simulink model "Projet_Final"  (R2024a)
settings: Solver=FixedStepAuto  StartTime=0.0  StopTime=6  FixedStep=Ts  RelTol=1e-3
values from neighbouring files (symbols this model uses):
  A1 = 0.548    [Parameters.m]
  A2 = 116    [Parameters.m]
  A3 = 0.4    [Parameters.m]
  A4 = 5    [Parameters.m]
  A5 = -21    [Parameters.m]
  A6 = 0.0068    [Parameters.m]
  C_Bat = 1e-3    (= 0.001)    [Parameters.m]    (also in Params_Battery_converter.m)
  C_dc = 4.5e-3    (= 0.0045)    [Parameters.m]
  f = 50    [Parameters.m]
  F = 0.0004924    [Parameters.m]
  G = 6.24    [Parameters.m]
  J = J_PMSG    (= 0.2227)    [Parameters.m]
  J_PMSG = 0.2227    [Parameters.m]
  ki_Ibat = 550    [Parameters.m]    (also in Params_Battery_converter.m)
  ki_id_grid = 225    [Parameters.m]
  ki_iq_grid = ki_id_grid    (= 225)    [Parameters.m]
  ki_isd = 13800    [Parameters.m]
  ki_omega = 0.6873    [Parameters.m]
  ki_PLL = 3200    [Parameters.m]
  ki_Q = 0.05    [Parameters.m]
  ki_vdc = C_dc * W_vdc^2    (= 28.8)    [Parameters.m]
  kp_Ibat = 6.28    [Parameters.m]    (also in Params_Battery_converter.m)
  kp_id_grid = 4.5    [Parameters.m]
  kp_iq_grid = kp_id_grid    (= 4.5)    [Parameters.m]
  kp_isd = 2.75    [Parameters.m]
  kp_omega = 3.108    [Parameters.m]
  kp_PLL = 180    [Parameters.m]
  kp_Q = 0.0005    [Parameters.m]
  kp_vdc = 2 * C_dc * W_vdc    (= 0.72)    [Parameters.m]
  Kt = 1.5 * p * Phi_r    (= 0.7164)    [Parameters.m]
  L_Bat = 2e-3    (= 0.002)    [Parameters.m]    (also in Params_Battery_converter.m)
  Lf = 8e-3    (= 0.008)    [Parameters.m]
  Ls = 0.000395    [Parameters.m]
  p = 4    [Parameters.m]
  Phi_r = 0.1194    [Parameters.m]
  R = 3.96    [Parameters.m]
  Rf = 0.01    [Parameters.m]
  rho = 1.225    [Parameters.m]
  Rs = 0.0485    [Parameters.m]
  S = pi*R^2    (= 49.2651993565)    [Parameters.m]
  Ts = 1e-6    (= 1e-06)    [Parameters.m]
  Vdc_ref = 700    [Parameters.m]    (also in Params_Battery_converter.m)
undefined symbols (not defined in the file or in its folder): Ion, Lithium
libraries: spsSeriesRLCBranchLib x19, slpidlib x11, spsMeanLib x6, spsThreePhaseVIMeasurementLib x6, spsThreePhaseBreakerLib x6, spsIdealSwitchLib x4, spsThreePhaseParallelRLCLoadLib x4, spsCurrentMeasurementLib x3, eeTransforms x3, spsPWMGenerator2LevelLib x3, spsVoltageMeasurementLib x3, spsUniversalBridgeLib x2
(part 2 of 3)

== system Projet_Final/Bidirectional DC–DC Converter/Battery Controller ==
  V_bat : Inport
  I_bat : Inport  Port=2
  P1 : Inport  Port=3
  P2 : Inport  Port=4
  Add2 : Sum  Inputs=+-
  Boucle I_bat : Scope  NumInputPorts=2
  Divide : Product  Inputs=*/
  PID Controller3 : slpidlib/PID Controller  Controller=PID  Form=Parallel  TimeDomain=Continuous-time  UseExternalTs=off  SampleTime=-1  IntegratorMethod=Forward Euler  FilterMethod=Forward Euler  ControllerParametersSource=internal  P=kp_Ibat  I=ki_Ibat  UseKiTs=off  D=0  UseExternalDerivativeSource=off  N=100  UseFilter=on  TunerSelectOption=Transfer Function Based (PID Tuner App)  InitialConditionSource=internal  InitialConditionForIntegrator=0  InitialConditionForFilter=0  DifferentiatorICPrevScaledInput=0  ExternalReset=none  TrackingMode=off  Kt=1  LimitOutput=off  SatLimitsSource=internal  UpperSaturationLimit=inf  LowerSaturationLimit=-inf  LinearizeAsGain=off  AntiWindupMode=none  Kb=1  LimitIntegrator=off  UpperIntegratorSaturationLimit=inf  LowerIntegratorSaturationLimit=-inf  POutMin=[]  POutMax=[]  IOutMin=[]  IOutMax=[]  DOutMin=[]  DOutMax=[]  NOutMin=[]  NOutMax=[]  SumOutMin=[]  SumOutMax=[]  SaturationOutMin=[]  SaturationOutMax=[]  PParamMin=[]  PParamMax=[]  IParamMin=[]  IParamMax=[]  DParamMin=[]  DParamMax=[]  NParamMin=[]  NParamMax=[]  KbParamMin=[]  KbParamMax=[]  KtParamMin=[]  KtParamMax=[]  KbOutMin=[]  KbOutMax=[]  KtOutMin=[]  KtOutMax=[]  IntegratorOutMin=[]  IntegratorOutMax=[]  FilterOutMin=[]  FilterOutMax=[]  SumI1OutMin=[]  SumI1OutMax=[]  SumI2OutMin=[]  SumI2OutMax=[]  SumI3OutMin=[]  SumI3OutMax=[]  SumI4OutMin=[]  SumI4OutMax=[]  SumDOutMin=[]  SumDOutMax=[]  DifferentiatorOutMin=[]  DifferentiatorOutMax=[]  FilterDiffOutCoefMin=[]  FilterDiffOutCoefMax=[]  ReciprocalOutMin=[]  ReciprocalOutMax=[]  SumDenOutMin=[]  SumDenOutMax=[]  SumNumOutMin=[]  SumNumOutMax=[]  DivideOutMin=[]  DivideOutMax=[]  UdiffTsProdOutMin=[]  UdiffTsProdOutMax=[]  NTsProdOutMin=[]  NTsProdOutMax=[]  UintegralTsProdOutMin=[]  UintegralTsProdOutMax=[]  UngainTsProdOutMin=[]  UngainTsProdOutMax=[]  ClampingZeroOutDataTypeStr=Inherit: Inherit via back propagation  ClampingZeroOutMin=[]  ClampingZeroOutMax=[]  FilterDenConstantOutDataTypeStr=Inherit: Inherit via back propagation  FilterDenConstantOutMin=[]  FilterDenConstantOutMax=[]  PCopyOutDataTypeStr=Inherit: Inherit via back propagation  PCopyOutMin=[]  PCopyOutMax=[]  NCopyOutDataTypeStr=Inherit: Inherit via back propagation  NCopyOutMin=[]  NCopyOutMax=[]  IntegratorContinuousStateAttributes=''  IntegratorStateMustResolveToSignalObject=off  IntegratorRTWStateStorageClass=Auto  FilterContinuousStateAttributes=''  FilterStateMustResolveToSignalObject=off  FilterRTWStateStorageClass=Auto  ParallelPVariant=InternalParameters  IdealPVariant=Disabled  IVariant=InternalParameters  DVariant=InternalParameters  IntegratorVariant=Continuous  SatVariant=Disabled  AWVariant=Passthrough  PCopyVariant=Disabled  TRVariant=Disabled  FdbkBlocksVariant=Forward  IdealPFdbkVariant=Disabled  SatFdbkVariant=Disabled  DerivativeFilterVariant=ContFilter  NVariant=InternalParameters  NCopyVariant=Disabled  FilterICVariant=InternalICsFilter  IntegratorICVariant=InternalICs  ExternalResetVariant=Disabled  TRSumVariant=Passthrough  SumFdbkVariant=Disabled  SumVariant=Sum_PID  TsampFilterVariant=InternalTs  TsampNgainVariant=Passthrough  TsampIntegralVariant=Disabled_SignalSpec  ExternalSaturationOutDataTypeStr=Inherit: Same as second input  DerivativeSourceVariant=ErrorSignal
  PWM Generator_ Single phase Half Bridge : Subsystem
  Saturation1 : Saturate  UpperLimit=700  LowerLimit=0.001
  Sum : Sum  Inputs=-+|
  Transfer Fcn3 : TransferFcn  Denominator=[1e-6 1]
  Transfer Fcn4 : TransferFcn  Denominator=[1e-6 1]
  PWM_1 : Outport  OutputWhenDisabled=reset  InitialOutput=0  VectorParamsAs1DForOutWhenUnconnected=off
  PWM_2 : Outport  Port=2  OutputWhenDisabled=reset  InitialOutput=0  VectorParamsAs1DForOutWhenUnconnected=off
  wires:
  I_bat/1 -> Transfer Fcn4/1
  PWM Generator_ Single phase Half Bridge/1(Buck) -> PWM_1/1
  PWM Generator_ Single phase Half Bridge/2(Boost) -> PWM_2/1
  PID Controller3/1 -> PWM Generator_ Single phase Half Bridge/1(err_filter)
  Sum/1 -> Transfer Fcn3/1
  Divide/1 -> Sum/2, Boucle I_bat/1
  Transfer Fcn3/1 -> PID Controller3/1
  Transfer Fcn4/1 -> Sum/1, Boucle I_bat/2
  Saturation1/1 -> Divide/2
  Add2/1 -> Divide/1
  V_bat/1 -> Saturation1/1
  P1/1 -> Add2/1
  P2/1 -> Add2/2

== system Projet_Final/Residential Load/Subsystem ==
  Constant2 : Constant
  Step : Step  Time=2  SampleTime=0
  Step1 : Step  Time=4  SampleTime=0
  tag scope: Charge1_ON=global, Charge2_ON=global, Charge3_ON=global
  wires:
  Constant2/1 -> [Charge1_ON]
  Step/1 -> [Charge2_ON]
  Step1/1 -> [Charge3_ON]

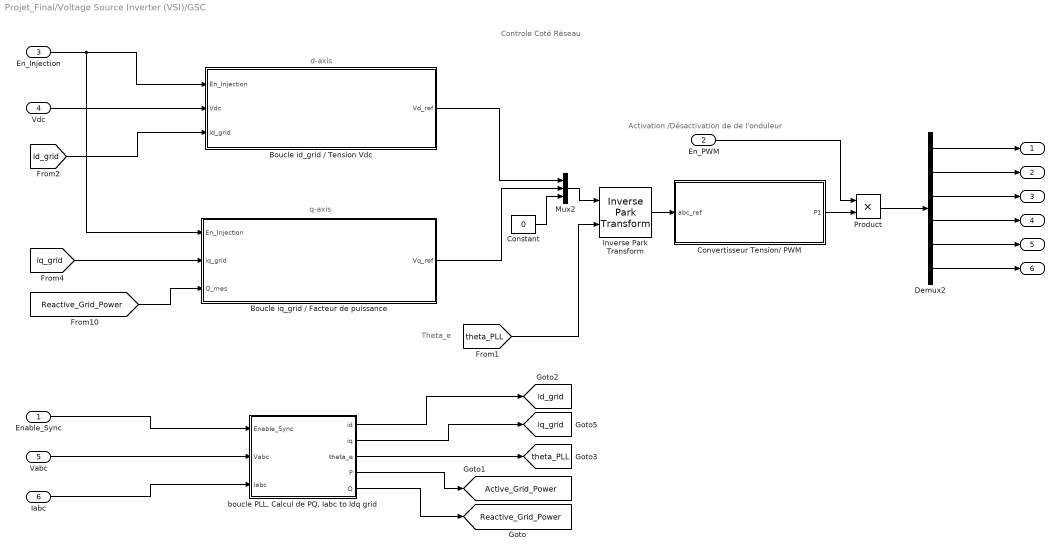
== system Projet_Final/Voltage Source Inverter (VSI)/GSC ==
  note: Controle Coté Réseau
  note: Activation /Désactivation de de l'onduleur
  note: d-axis
  note: Theta_e
  note: q-axis
  Enable_Sync : Inport
  En_PWM : Inport  Port=2
  En_Injection : Inport  Port=3
  Vdc : Inport  Port=4
  Vabc : Inport  Port=5
  Iabc : Inport  Port=6
  Boucle id_grid / Tension Vdc : Subsystem
  Boucle iq_grid / Facteur de puissance : Subsystem
  Constant : Constant  Value=0
  "Convertisseur Tension/ PWM " : Subsystem
  Demux2 : Demux  Outputs=6
  Inverse Park Transform : eeTransforms/Inverse Park Transform  AxisAlignment=Q-axis  PowerInvariant=off
      settings: LibrarySourceBlock=|
      | ee_sl_lib/Mathematical
      | Transforms/Inverse
      | Park Transform
  Mux2 : Mux  Inputs=3
  Product : Product
  "boucle PLL, Calcul de PQ, Iabc to Idq grid" : Subsystem
  " " : Outport
  "  " : Outport  Port=2
  "   " : Outport  Port=3
  "    " : Outport  Port=4
  "     " : Outport  Port=5
  "      " : Outport  Port=6
  tag scope: Active_Grid_Power=global, Reactive_Grid_Power=global, id_grid=global, iq_grid=global, theta_PLL=global
  wires:
  Mux2/1 -> Inverse Park Transform/1
  Constant/1 -> Mux2/3
  Inverse Park Transform/1 -> "Convertisseur Tension/ PWM "/1(abc_ref)
  Boucle iq_grid / Facteur de puissance/1(Vq_ref) -> Mux2/2
  Boucle id_grid / Tension Vdc/1(Vd_ref) -> Mux2/1
  Demux2/6 -> "      "/1
  Product/1 -> Demux2/1
  Demux2/3 -> "   "/1
  Demux2/5 -> "     "/1
  Demux2/1 -> " "/1
  Demux2/4 -> "    "/1
  Demux2/2 -> "  "/1
  "Convertisseur Tension/ PWM "/1(P1) -> Product/2
  Vdc/1 -> Boucle id_grid / Tension Vdc/2(Vdc)
  [id_grid] -> Boucle id_grid / Tension Vdc/3(id_grid)
  [Reactive_Grid_Power] -> Boucle iq_grid / Facteur de puissance/3(Q_mes)
  [iq_grid] -> Boucle iq_grid / Facteur de puissance/2(iq_grid)
  [theta_PLL] -> Inverse Park Transform/2
  Vabc/1 -> "boucle PLL, Calcul de PQ, Iabc to Idq grid"/2(Vabc)
  Iabc/1 -> "boucle PLL, Calcul de PQ, Iabc to Idq grid"/3(Iabc)
  "boucle PLL, Calcul de PQ, Iabc to Idq grid"/5(Q) -> [Reactive_Grid_Power]
  "boucle PLL, Calcul de PQ, Iabc to Idq grid"/4(P) -> [Active_Grid_Power]
  "boucle PLL, Calcul de PQ, Iabc to Idq grid"/1(id) -> [id_grid]
  "boucle PLL, Calcul de PQ, Iabc to Idq grid"/2(iq) -> [iq_grid]
  "boucle PLL, Calcul de PQ, Iabc to Idq grid"/3(theta_e) -> [theta_PLL]
  En_PWM/1 -> Product/1
  En_Injection/1 -> Boucle iq_grid / Facteur de puissance/1(En_Injection), Boucle id_grid / Tension Vdc/1(En_Injection)
  Enable_Sync/1 -> "boucle PLL, Calcul de PQ, Iabc to Idq grid"/1(Enable_Sync)

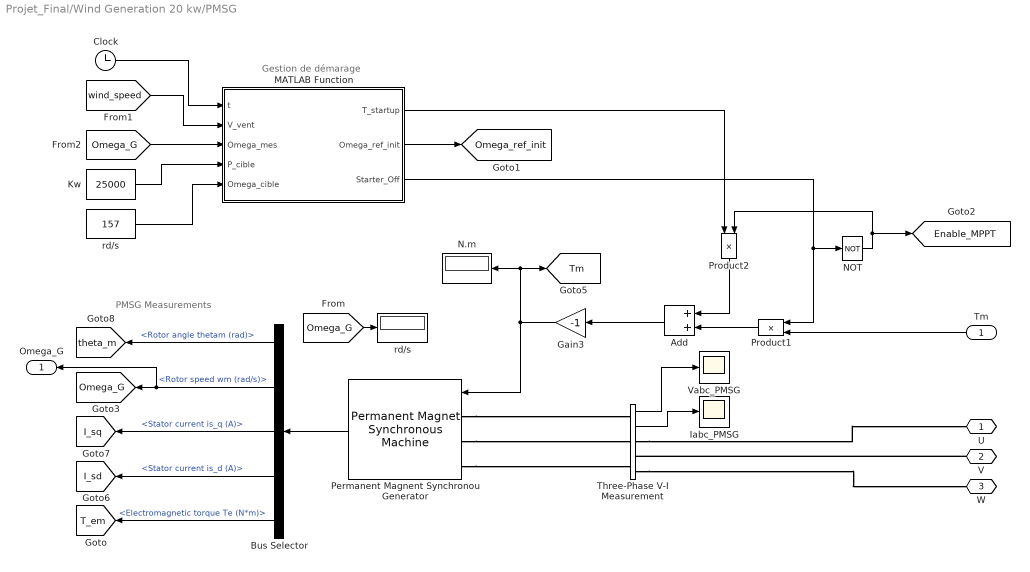
== system Projet_Final/Wind Generation 20 kw/PMSG ==
  note: Gestion de démarage
  note: PMSG Measurements
  Tm : Inport
  Add : Sum
  Bus Selector : BusSelector  OutputSignals=Rotor angle thetam (rad),Rotor speed wm (rad/s),Stator current is_q (A),Stator current is_d (A),Electromagnetic torque Te (N*m)
  Clock : Clock
  Gain3 : Gain  Gain=-1
  Iabc_PMSG : Scope
  Kw : Constant  Value=25000
  MATLAB Function : MATLAB Function  TreatAsAtomicUnit=on  SystemSampleTime=Ts
  N.m : Display
      settings: Format=bank
  NOT : Logic  Operator=NOT  IconShape=distinctive  AllPortsSameDT=off  OutDataTypeStr=boolean
  Permanent Magnent Synchronou Generator : spsPermanentMagnetSynchronousMachineLib/Permanent Magnet Synchronous Machine  NbPhases=3  FluxDistribution=Sinusoidal  RotorType=Round  MechanicalLoad=Torque Tm  PresetModel=No  ShowDetailedParameters=on  MeasurementBus=off  Resistance=Rs  Inductance=8.5e-3  dqInductances=[8.5e-3,8.5e-3]  La=Ls  MachineConstant=Flux linkage established by magnets (V.s)  Flux=Phi_r  VoltageCst=86.6271  TorqueCst=0.7164  Flat=120  Mechanical=[J F p 0]  PolePairs=4  InitialConditions=[0.01 ,0, 0,0]  InitialConditions5ph=[0 0 0 0 0 0]  RefAngle=90 degrees behind phase A axis (modified Park)  IterativeDiscreteModel=Trapezoidal non iterative  TsBlock=-1  TsPowergui=0
  Product1 : Product
  Product2 : Product
  Three-Phase V-I Measurement : spsThreePhaseVIMeasurementLib/Three-Phase V-I Measurement  VoltageMeasurement=phase-to-ground  SetLabelV=off  LabelV=Vabc  Vpu=off  VpuLL=off  CurrentMeasurement=yes  SetLabelI=off  LabelI=Iabc  Ipu=off  Pbase=100e6  Vbase=500e3  OutputType=Complex  PhasorSimulation=off  PSBequivalent=0
  Vabc_PMSG : Scope
  rd/s : Display
      settings: Format=bank
  "rd/s " : Constant  Value=157
  U : PMIOPort  Side=Right
  V : PMIOPort  Port=2  Side=Right
  W : PMIOPort  Port=3  Side=Right
  Omega_G : Outport
  tag scope: Enable_MPPT=global, I_sd=global, I_sq=global, Omega_G=global, Omega_ref_init=global, T_em=global, Tm=global, theta_m=global
  wires:
  Bus Selector/1 -> [theta_m]  "<Rotor angle thetam (rad)>"
  Bus Selector/2 -> Omega_G/1, [Omega_G]  "<Rotor speed wm (rad/s)>"
  Permanent Magnent Synchronou Generator/1 -> Bus Selector/1
  Bus Selector/4 -> [I_sd]  "<Stator current is_d (A)>"
  Bus Selector/5 -> [T_em]  "<Electromagnetic torque Te (N*m)>"
  Bus Selector/3 -> [I_sq]  "<Stator current is_q (A)>"
  Three-Phase V-I Measurement/1 -> Vabc_PMSG/1
  Three-Phase V-I Measurement/2 -> Iabc_PMSG/1
  Product1/1 -> Add/2
  MATLAB Function/3(Starter_Off) -> Product1/1, NOT/1
  MATLAB Function/2(Omega_ref_init) -> [Omega_ref_init]
  MATLAB Function/1(T_startup) -> Product2/1
  [Omega_G] -> MATLAB Function/3(Omega_mes)
  NOT/1 -> [Enable_MPPT], Product2/2
  [wind_speed] -> MATLAB Function/2(V_vent)
  Product2/1 -> Add/1
  Kw/1 -> MATLAB Function/4(P_cible)
  "rd/s "/1 -> MATLAB Function/5(Omega_cible)
  Clock/1 -> MATLAB Function/1(t)
  Add/1 -> Gain3/1
  Tm/1 -> Product1/2
  [Omega_G] -> rd/s/1
  Gain3/1 -> Permanent Magnent Synchronou Generator/1, [Tm], N.m/1
  connections:
  Permanent Magnent Synchronou Generator/LConn1 -- Three-Phase V-I Measurement/LConn1
  Permanent Magnent Synchronou Generator/LConn2 -- Three-Phase V-I Measurement/LConn2
  Permanent Magnent Synchronou Generator/LConn3 -- Three-Phase V-I Measurement/LConn3
  Three-Phase V-I Measurement/RConn1 -- U/RConn1
  V/RConn1 -- Three-Phase V-I Measurement/RConn2
  Three-Phase V-I Measurement/RConn3 -- W/RConn1

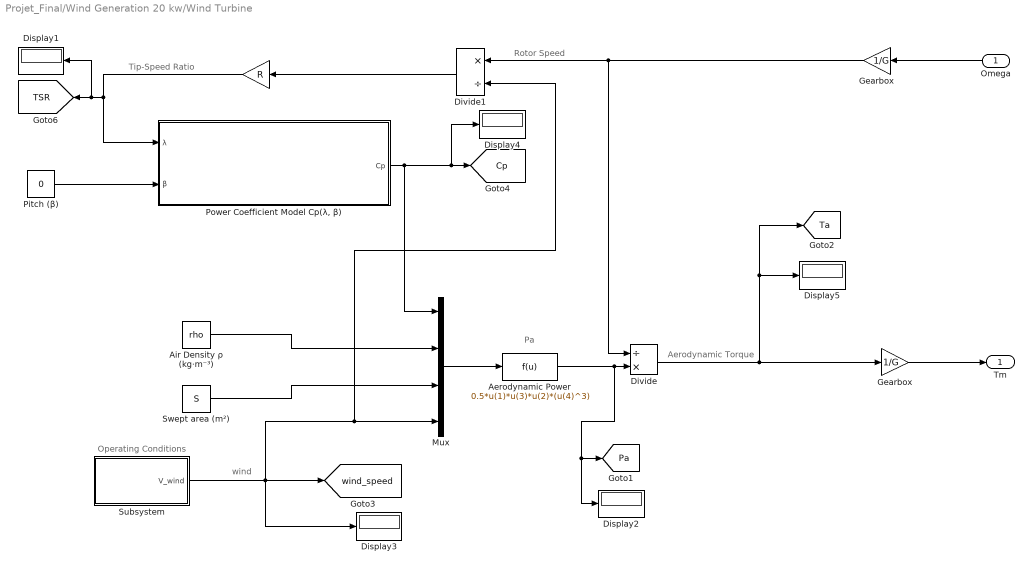
== system Projet_Final/Wind Generation 20 kw/Wind Turbine ==
  note: wind
  note: Rotor Speed
  note: Aerodynamic Torque
  note: Pa
  note: Operating Conditions
  note: Tip-Speed Ratio
  Omega : Inport
  "   " : Gain  Gain=R
  "Aerodynamic Power " : Fcn  Expr=0.5*u(1)*u(3)*u(2)*(u(4)^3)
  Air Density ρ (kg·m⁻³) : Constant  Value=rho
  Display{1..5} (5 alike) : Display
      settings: Format=bank
  Divide : Product  Inputs=/*
  Divide1 : Product  Inputs=*/
  Gearbox : Gain  Gain=1/G
  "Gearbox   " : Gain  Gain=1/G
  Mux : Mux
  "Pitch (β) " : Constant  Value=0
  "Power Coefficient Model Cp(λ, β)" : Subsystem
  Subsystem : Subsystem
  Swept area (m²) : Constant  Value=S
  Tm : Outport
  tag scope: Cp=global, Pa=global, TSR=global, Ta=global, wind_speed=global
  wires:
  Swept area (m²)/1 -> Mux/3
  "Power Coefficient Model Cp(λ, β)"/1(Cp) -> Display4/1, [Cp], Mux/1
  Subsystem/1(V_wind) -> Divide1/2, Mux/4, [wind_speed], Display3/1
  "Pitch (β) "/1 -> "Power Coefficient Model Cp(λ, β)"/2(β)
  Gearbox/1 -> Divide1/1, Divide/1
  Air Density ρ (kg·m⁻³)/1 -> Mux/2
  "   "/1 -> "Power Coefficient Model Cp(λ, β)"/1(λ), Display1/1, [TSR]
  Divide1/1 -> "   "/1
  Mux/1 -> "Aerodynamic Power "/1
  "Aerodynamic Power "/1 -> Display2/1, [Pa], Divide/2
  Divide/1 -> [Ta], Display5/1, "Gearbox   "/1
  "Gearbox   "/1 -> Tm/1
  Omega/1 -> Gearbox/1

== system Projet_Final/Active Rectifier/MSC/PWM Generation ==
  abc_ref : Inport
  Divide3 : Product  Inputs=*/
  PWM Generator (2-Level) : spsPWMGenerator2LevelLib/PWM Generator (2-Level)  ModulatorType=Three-phase bridge (6 pulses)  ModulatorMode=Unsynchronized  Fc=Fc  Pc=90  nF=27  MinMax="[ -1  1 ]"  SamplingTechnique=Natural  ModulatingSignals=off  m=0.8  Freq=60  Phase=0  Ts=Ts  ShowCarrierOutport=off
  Scope : Scope
  Unit Delay1 : UnitDelay  SampleTime=Ts  HasFrameUpgradeWarning=on
  indiceM=33_(1/(fr*33)3 : Constant  Value=Vdc_ref/2
  Commandes de Redresseur : Outport
  wires:
  indiceM=33_(1/(fr*33)3/1 -> Divide3/2
  abc_ref/1 -> Divide3/1
  PWM Generator (2-Level)/1 -> Commandes de Redresseur/1
  Unit Delay1/1 -> PWM Generator (2-Level)/1, Scope/1
  Divide3/1 -> Unit Delay1/1

== system Projet_Final/Active Rectifier/MSC/d-axis current controller with cross-coupling compensation ==
  note: isd_ref
  I_sd : Inport
  " Vd/Vdref" : Scope
  Constant : Constant  Value=0
  Decoupling Feedforward Terms : Subsystem
      settings: PortSchema="{\"entries\":[{\"content\":{\"sides\":[{\"content\":{\"connectorIds\":[\"In1\"]},\"type\":\"ConnectorPlacement.EquallySpacedRectSide\",\"uuid\":\"a35b541f-6c91-4579-89f1-6689e9beed7f\"},{\"content\":{\"connectorIds\":[\"Out1\"],\"side\":\"RIGHT\"},\"type\":\"ConnectorPlacement.EquallySpacedRectSide\",\"uuid\":\"c874527c-990c-4788-aa16-7f8a0c94d194\"},{\"content\":{\"side\":\"TOP\"},\"type\":\"ConnectorPlacement.EquallySpacedRectSide\",\"uuid\":\"b0161d26-106e-466a-8756-17981005591c\"},{\"content\":{\"connectorIds\":[\"In2\",\"In3\"],\"side\":\"BOTTOM\"},\"type\":\"ConnectorPlacement.EquallySpacedRectSide\",\"uuid\":\"87eba4bb-8cc6-4d91-843e-d033b71d377b\"}]},\"type\":\"ConnectorPlacement.EquallySpacedConnector\",\"uuid\":\"031ea5bd-d22b-4033-942a-a77822380b2b\"}],\"packageUris\":[\"http://schema.mathworks.com/mf0/Connector/R2020b\"],\"version\":\"1.0\"}"
  Mux1 : Mux  Inputs=2
  Mux2 : Mux  Inputs=2
  Sum : Sum  Inputs=+-
  Transfer Fcn{1..4} (4 alike) : TransferFcn  Denominator=[0.00004 1]
  d-axis Current Control Loop : Scope
  d-axis Current PI Controller : slpidlib/PID Controller  Controller=PI  Form=Parallel  TimeDomain=Continuous-time  UseExternalTs=off  SampleTime=Ts  IntegratorMethod=Forward Euler  FilterMethod=Forward Euler  ControllerParametersSource=internal  P=kp_isd  I=ki_isd  UseKiTs=off  D=0  UseExternalDerivativeSource=off  N=100  UseFilter=on  TunerSelectOption=Transfer Function Based (PID Tuner App)  InitialConditionSource=internal  InitialConditionForIntegrator=0  InitialConditionForFilter=0  DifferentiatorICPrevScaledInput=0  ExternalReset=none  TrackingMode=off  Kt=1  LimitOutput=off  SatLimitsSource=internal  UpperSaturationLimit=inf  LowerSaturationLimit=-inf  LinearizeAsGain=on  AntiWindupMode=none  Kb=1  LimitIntegrator=off  UpperIntegratorSaturationLimit=inf  LowerIntegratorSaturationLimit=-inf  POutMin=[]  POutMax=[]  IOutMin=[]  IOutMax=[]  DOutMin=[]  DOutMax=[]  NOutMin=[]  NOutMax=[]  SumOutMin=[]  SumOutMax=[]  SaturationOutMin=[]  SaturationOutMax=[]  PParamMin=[]  PParamMax=[]  IParamMin=[]  IParamMax=[]  DParamMin=[]  DParamMax=[]  NParamMin=[]  NParamMax=[]  KbParamMin=[]  KbParamMax=[]  KtParamMin=[]  KtParamMax=[]  KbOutMin=[]  KbOutMax=[]  KtOutMin=[]  KtOutMax=[]  IntegratorOutMin=[]  IntegratorOutMax=[]  FilterOutMin=[]  FilterOutMax=[]  SumI1OutMin=[]  SumI1OutMax=[]  SumI2OutMin=[]  SumI2OutMax=[]  SumI3OutMin=[]  SumI3OutMax=[]  SumI4OutMin=[]  SumI4OutMax=[]  SumDOutMin=[]  SumDOutMax=[]  DifferentiatorOutMin=[]  DifferentiatorOutMax=[]  FilterDiffOutCoefMin=[]  FilterDiffOutCoefMax=[]  ReciprocalOutMin=[]  ReciprocalOutMax=[]  SumDenOutMin=[]  SumDenOutMax=[]  SumNumOutMin=[]  SumNumOutMax=[]  DivideOutMin=[]  DivideOutMax=[]  UdiffTsProdOutMin=[]  UdiffTsProdOutMax=[]  NTsProdOutMin=[]  NTsProdOutMax=[]  UintegralTsProdOutMin=[]  UintegralTsProdOutMax=[]  UngainTsProdOutMin=[]  UngainTsProdOutMax=[]  ClampingZeroOutDataTypeStr=Inherit: Inherit via back propagation  ClampingZeroOutMin=[]  ClampingZeroOutMax=[]  FilterDenConstantOutDataTypeStr=Inherit: Inherit via back propagation  FilterDenConstantOutMin=[]  FilterDenConstantOutMax=[]  PCopyOutDataTypeStr=Inherit: Inherit via back propagation  PCopyOutMin=[]  PCopyOutMax=[]  NCopyOutDataTypeStr=Inherit: Inherit via back propagation  NCopyOutMin=[]  NCopyOutMax=[]  IntegratorContinuousStateAttributes=''  IntegratorStateMustResolveToSignalObject=off  IntegratorRTWStateStorageClass=Auto  FilterContinuousStateAttributes=''  FilterStateMustResolveToSignalObject=off  FilterRTWStateStorageClass=Auto  ParallelPVariant=InternalParameters  IdealPVariant=Disabled  IVariant=InternalParameters  DVariant=Disabled  IntegratorVariant=Continuous  SatVariant=Disabled  AWVariant=Passthrough  PCopyVariant=Disabled  TRVariant=Disabled  FdbkBlocksVariant=Forward  IdealPFdbkVariant=Disabled  SatFdbkVariant=Disabled  DerivativeFilterVariant=Disabled  NVariant=Disabled  NCopyVariant=Disabled_SignalSpec  FilterICVariant=Disabled  IntegratorICVariant=InternalICs  ExternalResetVariant=Disabled  TRSumVariant=Passthrough  SumFdbkVariant=Disabled  SumVariant=Sum_PI  TsampFilterVariant=InternalTs  TsampNgainVariant=Passthrough  TsampIntegralVariant=Disabled_SignalSpec  ExternalSaturationOutDataTypeStr=Inherit: Same as second input  DerivativeSourceVariant=Disabled
  Vd_ref : Outport
  wires:
  I_sd/1 -> Transfer Fcn4/1
  [I_sq] -> Transfer Fcn2/1
  [Omega_G] -> Decoupling Feedforward Terms/3(Wm)
  Mux1/1 -> d-axis Current Control Loop/1
  Constant/1 -> Sum/1, Mux1/2
  Sum/1 -> Transfer Fcn3/1
  Decoupling Feedforward Terms/1(Vdref) -> Mux2/2, Vd_ref/1
  d-axis Current PI Controller/1 -> Transfer Fcn1/1, Mux2/1
  Transfer Fcn2/1 -> Decoupling Feedforward Terms/2(Iq)
  Mux2/1 -> " Vd/Vdref"/1
  Transfer Fcn3/1 -> d-axis Current PI Controller/1
  Transfer Fcn1/1 -> Decoupling Feedforward Terms/1(vd)
  Transfer Fcn4/1 -> Sum/2, Mux1/1

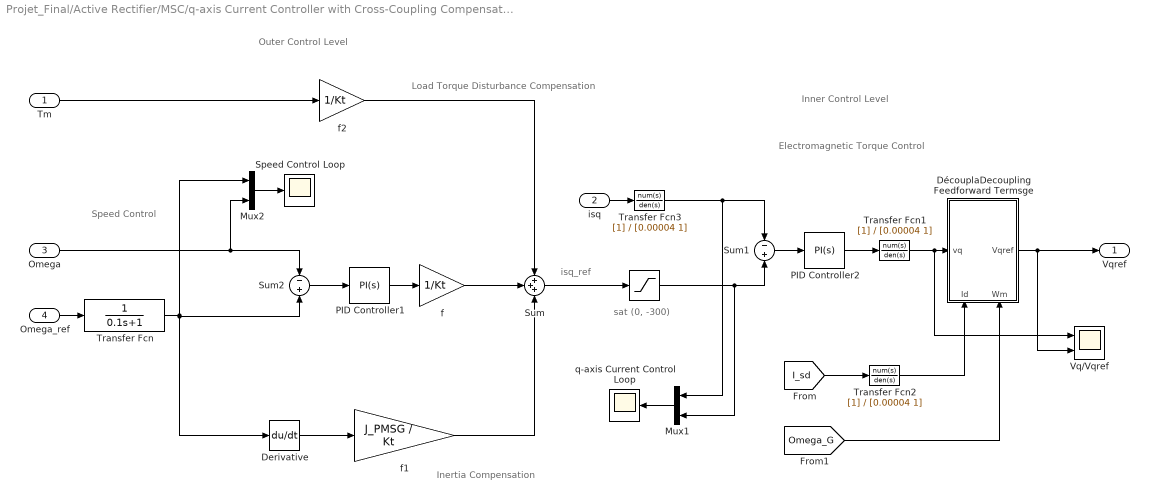
== system Projet_Final/Active Rectifier/MSC/q-axis Current Controller with Cross-Coupling Compensation  ==
  note: Speed Control
  note: sat (0, -300)
  note: Load Torque Disturbance Compensation
  note: isq_ref
  note: Inertia Compensation
  note: Electromagnetic Torque Control
  note: Inner Control Level
  note: Outer Control Level
  Tm : Inport
  isq : Inport  Port=2
  Omega : Inport  Port=3
  Omega_ref : Inport  Port=4
  "  " : Saturate  UpperLimit=0  LowerLimit=-300
  Derivative : Derivative
  DécouplaDecoupling Feedforward Termsge : Subsystem
      settings: PortSchema="{\"entries\":[{\"content\":{\"sides\":[{\"content\":{\"connectorIds\":[\"In1\"]},\"type\":\"ConnectorPlacement.EquallySpacedRectSide\",\"uuid\":\"a35b541f-6c91-4579-89f1-6689e9beed7f\"},{\"content\":{\"connectorIds\":[\"Out1\"],\"side\":\"RIGHT\"},\"type\":\"ConnectorPlacement.EquallySpacedRectSide\",\"uuid\":\"c874527c-990c-4788-aa16-7f8a0c94d194\"},{\"content\":{\"side\":\"TOP\"},\"type\":\"ConnectorPlacement.EquallySpacedRectSide\",\"uuid\":\"b0161d26-106e-466a-8756-17981005591c\"},{\"content\":{\"connectorIds\":[\"In2\",\"In3\"],\"side\":\"BOTTOM\"},\"type\":\"ConnectorPlacement.EquallySpacedRectSide\",\"uuid\":\"6bea0741-ba37-48dd-9c1f-2166530afd2a\"}]},\"type\":\"ConnectorPlacement.EquallySpacedConnector\",\"uuid\":\"031ea5bd-d22b-4033-942a-a77822380b2b\"}],\"packageUris\":[\"http://schema.mathworks.com/mf0/Connector/R2020b\"],\"version\":\"1.0\"}"
  Mux1 : Mux  Inputs=2
  Mux2 : Mux  Inputs=2
  PID Controller1 : slpidlib/PID Controller  Controller=PI  Form=Parallel  TimeDomain=Continuous-time  UseExternalTs=off  SampleTime=Ts  IntegratorMethod=Forward Euler  FilterMethod=Forward Euler  ControllerParametersSource=internal  P=kp_omega  I=ki_omega  UseKiTs=off  D=0  UseExternalDerivativeSource=off  N=100  UseFilter=on  TunerSelectOption=Transfer Function Based (PID Tuner App)  InitialConditionSource=internal  InitialConditionForIntegrator=0  InitialConditionForFilter=0  DifferentiatorICPrevScaledInput=0  ExternalReset=none  TrackingMode=off  Kt=1  LimitOutput=off  SatLimitsSource=internal  UpperSaturationLimit=222.3  LowerSaturationLimit=0  LinearizeAsGain=on  AntiWindupMode=back-calculation  Kb=1  LimitIntegrator=off  UpperIntegratorSaturationLimit=inf  LowerIntegratorSaturationLimit=-inf  POutMin=[]  POutMax=[]  IOutMin=[]  IOutMax=[]  DOutMin=[]  DOutMax=[]  NOutMin=[]  NOutMax=[]  SumOutMin=[]  SumOutMax=[]  SaturationOutMin=[]  SaturationOutMax=[]  PParamMin=[]  PParamMax=[]  IParamMin=[]  IParamMax=[]  DParamMin=[]  DParamMax=[]  NParamMin=[]  NParamMax=[]  KbParamMin=[]  KbParamMax=[]  KtParamMin=[]  KtParamMax=[]  KbOutMin=[]  KbOutMax=[]  KtOutMin=[]  KtOutMax=[]  IntegratorOutMin=[]  IntegratorOutMax=[]  FilterOutMin=[]  FilterOutMax=[]  SumI1OutMin=[]  SumI1OutMax=[]  SumI2OutMin=[]  SumI2OutMax=[]  SumI3OutMin=[]  SumI3OutMax=[]  SumI4OutMin=[]  SumI4OutMax=[]  SumDOutMin=[]  SumDOutMax=[]  DifferentiatorOutMin=[]  DifferentiatorOutMax=[]  FilterDiffOutCoefMin=[]  FilterDiffOutCoefMax=[]  ReciprocalOutMin=[]  ReciprocalOutMax=[]  SumDenOutMin=[]  SumDenOutMax=[]  SumNumOutMin=[]  SumNumOutMax=[]  DivideOutMin=[]  DivideOutMax=[]  UdiffTsProdOutMin=[]  UdiffTsProdOutMax=[]  NTsProdOutMin=[]  NTsProdOutMax=[]  UintegralTsProdOutMin=[]  UintegralTsProdOutMax=[]  UngainTsProdOutMin=[]  UngainTsProdOutMax=[]  ClampingZeroOutDataTypeStr=Inherit: Inherit via back propagation  ClampingZeroOutMin=[]  ClampingZeroOutMax=[]  FilterDenConstantOutDataTypeStr=Inherit: Inherit via back propagation  FilterDenConstantOutMin=[]  FilterDenConstantOutMax=[]  PCopyOutDataTypeStr=Inherit: Inherit via back propagation  PCopyOutMin=[]  PCopyOutMax=[]  NCopyOutDataTypeStr=Inherit: Inherit via back propagation  NCopyOutMin=[]  NCopyOutMax=[]  IntegratorContinuousStateAttributes=''  IntegratorStateMustResolveToSignalObject=off  IntegratorRTWStateStorageClass=Auto  FilterContinuousStateAttributes=''  FilterStateMustResolveToSignalObject=off  FilterRTWStateStorageClass=Auto  ParallelPVariant=InternalParameters  IdealPVariant=Disabled  IVariant=InternalParameters  DVariant=Disabled  IntegratorVariant=Continuous  SatVariant=Disabled  AWVariant=Passthrough  PCopyVariant=Disabled  TRVariant=Disabled  FdbkBlocksVariant=Forward  IdealPFdbkVariant=Disabled  SatFdbkVariant=Disabled  DerivativeFilterVariant=Disabled  NVariant=Disabled  NCopyVariant=Disabled_SignalSpec  FilterICVariant=Disabled  IntegratorICVariant=InternalICs  ExternalResetVariant=Disabled  TRSumVariant=Passthrough  SumFdbkVariant=Disabled  SumVariant=Sum_PI  TsampFilterVariant=InternalTs  TsampNgainVariant=Passthrough  TsampIntegralVariant=Disabled_SignalSpec  ExternalSaturationOutDataTypeStr=Inherit: Same as second input  DerivativeSourceVariant=Disabled
  PID Controller2 : slpidlib/PID Controller  Controller=PI  Form=Parallel  TimeDomain=Continuous-time  UseExternalTs=off  SampleTime=Ts  IntegratorMethod=Forward Euler  FilterMethod=Forward Euler  ControllerParametersSource=internal  P=kp_isd  I=ki_isd  UseKiTs=off  D=0  UseExternalDerivativeSource=off  N=100  UseFilter=on  TunerSelectOption=Transfer Function Based (PID Tuner App)  InitialConditionSource=internal  InitialConditionForIntegrator=0  InitialConditionForFilter=0  DifferentiatorICPrevScaledInput=0  ExternalReset=none  TrackingMode=off  Kt=1  LimitOutput=off  SatLimitsSource=internal  UpperSaturationLimit=inf  LowerSaturationLimit=-inf  LinearizeAsGain=on  AntiWindupMode=none  Kb=1  LimitIntegrator=off  UpperIntegratorSaturationLimit=inf  LowerIntegratorSaturationLimit=-inf  POutMin=[]  POutMax=[]  IOutMin=[]  IOutMax=[]  DOutMin=[]  DOutMax=[]  NOutMin=[]  NOutMax=[]  SumOutMin=[]  SumOutMax=[]  SaturationOutMin=[]  SaturationOutMax=[]  PParamMin=[]  PParamMax=[]  IParamMin=[]  IParamMax=[]  DParamMin=[]  DParamMax=[]  NParamMin=[]  NParamMax=[]  KbParamMin=[]  KbParamMax=[]  KtParamMin=[]  KtParamMax=[]  KbOutMin=[]  KbOutMax=[]  KtOutMin=[]  KtOutMax=[]  IntegratorOutMin=[]  IntegratorOutMax=[]  FilterOutMin=[]  FilterOutMax=[]  SumI1OutMin=[]  SumI1OutMax=[]  SumI2OutMin=[]  SumI2OutMax=[]  SumI3OutMin=[]  SumI3OutMax=[]  SumI4OutMin=[]  SumI4OutMax=[]  SumDOutMin=[]  SumDOutMax=[]  DifferentiatorOutMin=[]  DifferentiatorOutMax=[]  FilterDiffOutCoefMin=[]  FilterDiffOutCoefMax=[]  ReciprocalOutMin=[]  ReciprocalOutMax=[]  SumDenOutMin=[]  SumDenOutMax=[]  SumNumOutMin=[]  SumNumOutMax=[]  DivideOutMin=[]  DivideOutMax=[]  UdiffTsProdOutMin=[]  UdiffTsProdOutMax=[]  NTsProdOutMin=[]  NTsProdOutMax=[]  UintegralTsProdOutMin=[]  UintegralTsProdOutMax=[]  UngainTsProdOutMin=[]  UngainTsProdOutMax=[]  ClampingZeroOutDataTypeStr=Inherit: Inherit via back propagation  ClampingZeroOutMin=[]  ClampingZeroOutMax=[]  FilterDenConstantOutDataTypeStr=Inherit: Inherit via back propagation  FilterDenConstantOutMin=[]  FilterDenConstantOutMax=[]  PCopyOutDataTypeStr=Inherit: Inherit via back propagation  PCopyOutMin=[]  PCopyOutMax=[]  NCopyOutDataTypeStr=Inherit: Inherit via back propagation  NCopyOutMin=[]  NCopyOutMax=[]  IntegratorContinuousStateAttributes=''  IntegratorStateMustResolveToSignalObject=off  IntegratorRTWStateStorageClass=Auto  FilterContinuousStateAttributes=''  FilterStateMustResolveToSignalObject=off  FilterRTWStateStorageClass=Auto  ParallelPVariant=InternalParameters  IdealPVariant=Disabled  IVariant=InternalParameters  DVariant=Disabled  IntegratorVariant=Continuous  SatVariant=Disabled  AWVariant=Passthrough  PCopyVariant=Disabled  TRVariant=Disabled  FdbkBlocksVariant=Forward  IdealPFdbkVariant=Disabled  SatFdbkVariant=Disabled  DerivativeFilterVariant=Disabled  NVariant=Disabled  NCopyVariant=Disabled_SignalSpec  FilterICVariant=Disabled  IntegratorICVariant=InternalICs  ExternalResetVariant=Disabled  TRSumVariant=Passthrough  SumFdbkVariant=Disabled  SumVariant=Sum_PI  TsampFilterVariant=InternalTs  TsampNgainVariant=Passthrough  TsampIntegralVariant=Disabled_SignalSpec  ExternalSaturationOutDataTypeStr=Inherit: Same as second input  DerivativeSourceVariant=Disabled
  Speed Control Loop : Scope
  Sum : Sum  Inputs=+++
  Sum1 : Sum  Inputs=-+
  Sum2 : Sum  Inputs=-+
  Transfer Fcn : TransferFcn  Denominator=[0.1 1]
  Transfer Fcn1 : TransferFcn  Denominator=[0.00004 1]
  Transfer Fcn2 : TransferFcn  Denominator=[0.00004 1]
  Transfer Fcn3 : TransferFcn  Denominator=[0.00004 1]
  Vq/Vqref : Scope  NumInputPorts=2
  f : Gain  Gain=1/Kt  SaturateOnIntegerOverflow=on  OutDataTypeStr=Inherit: Same as input  ParamDataTypeStr=Inherit: Same as input
  f1 : Gain  Gain=J_PMSG / Kt  SaturateOnIntegerOverflow=on  OutDataTypeStr=Inherit: Same as input  ParamDataTypeStr=Inherit: Same as input
  f2 : Gain  Gain=1/Kt  SaturateOnIntegerOverflow=on  OutDataTypeStr=Inherit: Same as input  ParamDataTypeStr=Inherit: Same as input
  q-axis Current Control Loop : Scope
  Vqref : Outport
  wires:
  Mux1/1 -> q-axis Current Control Loop/1
  Omega/1 -> Mux2/2, Sum2/1
  isq/1 -> Transfer Fcn3/1
  PID Controller2/1 -> Transfer Fcn1/1
  Sum1/1 -> PID Controller2/1
  Sum2/1 -> PID Controller1/1
  Mux2/1 -> Speed Control Loop/1
  PID Controller1/1 -> f/1
  Tm/1 -> f2/1
  Derivative/1 -> f1/1
  DécouplaDecoupling Feedforward Termsge/1(Vqref) -> Vqref/1, Vq/Vqref/2
  Transfer Fcn2/1 -> DécouplaDecoupling Feedforward Termsge/2(Id)
  [Omega_G] -> DécouplaDecoupling Feedforward Termsge/3(Wm)
  "  "/1 -> Mux1/2, Sum1/2
  f/1 -> Sum/2
  Sum/1 -> "  "/1
  f2/1 -> Sum/1
  Transfer Fcn/1 -> Derivative/1, Sum2/2, Mux2/1
  Omega_ref/1 -> Transfer Fcn/1
  f1/1 -> Sum/3
  [I_sd] -> Transfer Fcn2/1
  Transfer Fcn1/1 -> Vq/Vqref/1, DécouplaDecoupling Feedforward Termsge/1(vq)
  Transfer Fcn3/1 -> Sum1/1, Mux1/1

== system Projet_Final/Bidirectional DC–DC Converter/Battery Controller/PWM Generator_ Single phase Half Bridge ==
  err_filter : Inport
  Add : Sum
  Constant : Constant  Value=-1
  Demux5 : Demux  Outputs=2
  Gain : Gain  Gain=2
  PWM Generator (2-Level) : spsPWMGenerator2LevelLib/PWM Generator (2-Level)  ModulatorType=Single-phase half-bridge (2 pulses)  ModulatorMode=Unsynchronized  Fc=Fc  Pc=90  nF=27  MinMax="[ -1  1 ]"  SamplingTechnique=Natural  ModulatingSignals=off  m=0.8  Freq=60  Phase=0  Ts=Ts  ShowCarrierOutport=off
  Buck : Outport
  Boost : Outport  Port=2
  wires:
  Constant/1 -> Add/2
  Gain/1 -> Add/1
  Demux5/2 -> Boost/1
  Add/1 -> PWM Generator (2-Level)/1  "duty_to_-1_1"
  err_filter/1 -> Gain/1
  Demux5/1 -> Buck/1
  PWM Generator (2-Level)/1 -> Demux5/1

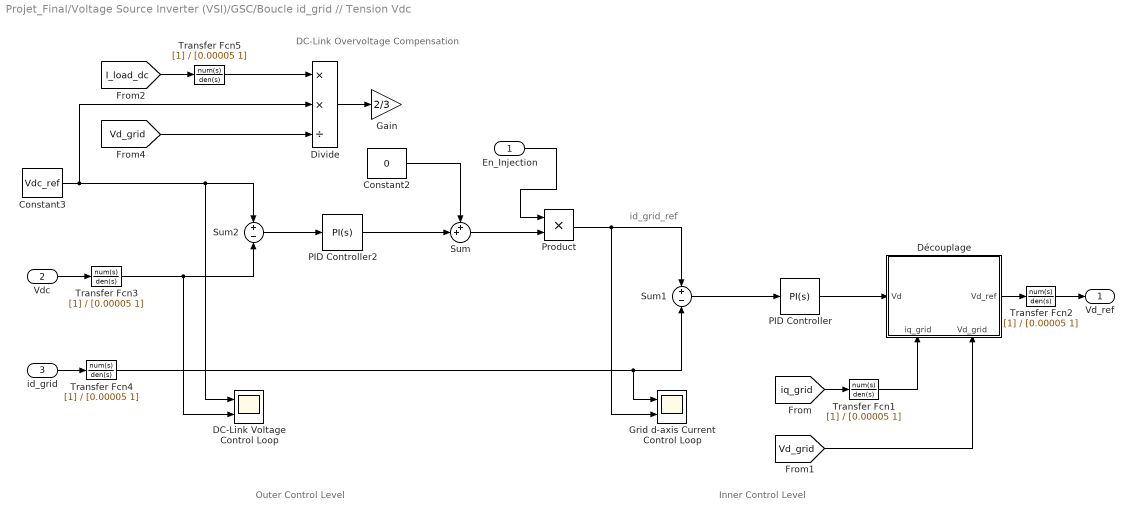
== system Projet_Final/Voltage Source Inverter (VSI)/GSC/Boucle id_grid // Tension Vdc ==
  note: Inner Control Level
  note: DC-Link Overvoltage Compensation
  note: id_grid_ref
  note: Outer Control Level
  En_Injection : Inport
  Vdc : Inport  Port=2
  id_grid : Inport  Port=3
  Constant2 : Constant  Value=0
  Constant3 : Constant  Value=Vdc_ref
  DC-Link Voltage Control Loop : Scope  NumInputPorts=2
  Divide : Product  Inputs=**/
  Découplage : Subsystem
      settings: PortSchema="{\"entries\":[{\"content\":{\"sides\":[{\"content\":{\"connectorIds\":[\"In1\"]},\"type\":\"ConnectorPlacement.EquallySpacedRectSide\",\"uuid\":\"7d3af298-2f9f-475a-a651-f5eac2186357\"},{\"content\":{\"connectorIds\":[\"Out1\"],\"side\":\"RIGHT\"},\"type\":\"ConnectorPlacement.EquallySpacedRectSide\",\"uuid\":\"aa22588b-a98c-4a55-adf5-26eaad5d3043\"},{\"content\":{\"side\":\"TOP\"},\"type\":\"ConnectorPlacement.EquallySpacedRectSide\",\"uuid\":\"895af8ff-ad69-460f-8331-727a35d5d5ec\"},{\"content\":{\"connectorIds\":[\"In2\",\"In3\"],\"side\":\"BOTTOM\"},\"type\":\"ConnectorPlacement.EquallySpacedRectSide\",\"uuid\":\"a79db6ec-2ceb-4bca-883f-aa3bf861af08\"}]},\"type\":\"ConnectorPlacement.EquallySpacedConnector\",\"uuid\":\"f85c84fc-5e67-455b-b890-ed27a42cb9c3\"}],\"packageUris\":[\"http://schema.mathworks.com/mf0/Connector/R2020b\"],\"version\":\"1.0\"}"
  Gain : Gain  Gain=2/3
  Grid d-axis Current Control Loop : Scope  NumInputPorts=2
  PID Controller : slpidlib/PID Controller  Controller=PI  Form=Parallel  TimeDomain=Continuous-time  UseExternalTs=off  SampleTime=-1  IntegratorMethod=Forward Euler  FilterMethod=Forward Euler  ControllerParametersSource=internal  P=kp_id_grid  I=ki_id_grid  UseKiTs=off  D=0  UseExternalDerivativeSource=off  N=100  UseFilter=on  TunerSelectOption=Transfer Function Based (PID Tuner App)  InitialConditionSource=internal  InitialConditionForIntegrator=0  InitialConditionForFilter=0  DifferentiatorICPrevScaledInput=0  ExternalReset=none  TrackingMode=off  Kt=1  LimitOutput=off  SatLimitsSource=internal  UpperSaturationLimit=inf  LowerSaturationLimit=-inf  LinearizeAsGain=on  AntiWindupMode=none  Kb=1  LimitIntegrator=off  UpperIntegratorSaturationLimit=inf  LowerIntegratorSaturationLimit=-inf  POutMin=[]  POutMax=[]  IOutMin=[]  IOutMax=[]  DOutMin=[]  DOutMax=[]  NOutMin=[]  NOutMax=[]  SumOutMin=[]  SumOutMax=[]  SaturationOutMin=[]  SaturationOutMax=[]  PParamMin=[]  PParamMax=[]  IParamMin=[]  IParamMax=[]  DParamMin=[]  DParamMax=[]  NParamMin=[]  NParamMax=[]  KbParamMin=[]  KbParamMax=[]  KtParamMin=[]  KtParamMax=[]  KbOutMin=[]  KbOutMax=[]  KtOutMin=[]  KtOutMax=[]  IntegratorOutMin=[]  IntegratorOutMax=[]  FilterOutMin=[]  FilterOutMax=[]  SumI1OutMin=[]  SumI1OutMax=[]  SumI2OutMin=[]  SumI2OutMax=[]  SumI3OutMin=[]  SumI3OutMax=[]  SumI4OutMin=[]  SumI4OutMax=[]  SumDOutMin=[]  SumDOutMax=[]  DifferentiatorOutMin=[]  DifferentiatorOutMax=[]  FilterDiffOutCoefMin=[]  FilterDiffOutCoefMax=[]  ReciprocalOutMin=[]  ReciprocalOutMax=[]  SumDenOutMin=[]  SumDenOutMax=[]  SumNumOutMin=[]  SumNumOutMax=[]  DivideOutMin=[]  DivideOutMax=[]  UdiffTsProdOutMin=[]  UdiffTsProdOutMax=[]  NTsProdOutMin=[]  NTsProdOutMax=[]  UintegralTsProdOutMin=[]  UintegralTsProdOutMax=[]  UngainTsProdOutMin=[]  UngainTsProdOutMax=[]  ClampingZeroOutDataTypeStr=Inherit: Inherit via back propagation  ClampingZeroOutMin=[]  ClampingZeroOutMax=[]  FilterDenConstantOutDataTypeStr=Inherit: Inherit via back propagation  FilterDenConstantOutMin=[]  FilterDenConstantOutMax=[]  PCopyOutDataTypeStr=Inherit: Inherit via back propagation  PCopyOutMin=[]  PCopyOutMax=[]  NCopyOutDataTypeStr=Inherit: Inherit via back propagation  NCopyOutMin=[]  NCopyOutMax=[]  IntegratorContinuousStateAttributes=''  IntegratorStateMustResolveToSignalObject=off  IntegratorRTWStateStorageClass=Auto  FilterContinuousStateAttributes=''  FilterStateMustResolveToSignalObject=off  FilterRTWStateStorageClass=Auto  ParallelPVariant=InternalParameters  IdealPVariant=Disabled  IVariant=InternalParameters  DVariant=Disabled  IntegratorVariant=Continuous  SatVariant=Disabled  AWVariant=Passthrough  PCopyVariant=Disabled  TRVariant=Disabled  FdbkBlocksVariant=Forward  IdealPFdbkVariant=Disabled  SatFdbkVariant=Disabled  DerivativeFilterVariant=Disabled  NVariant=Disabled  NCopyVariant=Disabled_SignalSpec  FilterICVariant=Disabled  IntegratorICVariant=InternalICs  ExternalResetVariant=Disabled  TRSumVariant=Passthrough  SumFdbkVariant=Disabled  SumVariant=Sum_PI  TsampFilterVariant=InternalTs  TsampNgainVariant=Passthrough  TsampIntegralVariant=Disabled_SignalSpec  ExternalSaturationOutDataTypeStr=Inherit: Same as second input  DerivativeSourceVariant=Disabled
  PID Controller2 : slpidlib/PID Controller  Controller=PI  Form=Parallel  TimeDomain=Continuous-time  UseExternalTs=off  SampleTime=-1  IntegratorMethod=Forward Euler  FilterMethod=Forward Euler  ControllerParametersSource=internal  P=kp_vdc  I=ki_vdc  UseKiTs=off  D=0  UseExternalDerivativeSource=off  N=100  UseFilter=on  TunerSelectOption=Transfer Function Based (PID Tuner App)  InitialConditionSource=internal  InitialConditionForIntegrator=0  InitialConditionForFilter=0  DifferentiatorICPrevScaledInput=0  ExternalReset=none  TrackingMode=off  Kt=1  LimitOutput=off  SatLimitsSource=internal  UpperSaturationLimit=inf  LowerSaturationLimit=-inf  LinearizeAsGain=on  AntiWindupMode=none  Kb=1  LimitIntegrator=off  UpperIntegratorSaturationLimit=inf  LowerIntegratorSaturationLimit=-inf  POutMin=[]  POutMax=[]  IOutMin=[]  IOutMax=[]  DOutMin=[]  DOutMax=[]  NOutMin=[]  NOutMax=[]  SumOutMin=[]  SumOutMax=[]  SaturationOutMin=[]  SaturationOutMax=[]  PParamMin=[]  PParamMax=[]  IParamMin=[]  IParamMax=[]  DParamMin=[]  DParamMax=[]  NParamMin=[]  NParamMax=[]  KbParamMin=[]  KbParamMax=[]  KtParamMin=[]  KtParamMax=[]  KbOutMin=[]  KbOutMax=[]  KtOutMin=[]  KtOutMax=[]  IntegratorOutMin=[]  IntegratorOutMax=[]  FilterOutMin=[]  FilterOutMax=[]  SumI1OutMin=[]  SumI1OutMax=[]  SumI2OutMin=[]  SumI2OutMax=[]  SumI3OutMin=[]  SumI3OutMax=[]  SumI4OutMin=[]  SumI4OutMax=[]  SumDOutMin=[]  SumDOutMax=[]  DifferentiatorOutMin=[]  DifferentiatorOutMax=[]  FilterDiffOutCoefMin=[]  FilterDiffOutCoefMax=[]  ReciprocalOutMin=[]  ReciprocalOutMax=[]  SumDenOutMin=[]  SumDenOutMax=[]  SumNumOutMin=[]  SumNumOutMax=[]  DivideOutMin=[]  DivideOutMax=[]  UdiffTsProdOutMin=[]  UdiffTsProdOutMax=[]  NTsProdOutMin=[]  NTsProdOutMax=[]  UintegralTsProdOutMin=[]  UintegralTsProdOutMax=[]  UngainTsProdOutMin=[]  UngainTsProdOutMax=[]  ClampingZeroOutDataTypeStr=Inherit: Inherit via back propagation  ClampingZeroOutMin=[]  ClampingZeroOutMax=[]  FilterDenConstantOutDataTypeStr=Inherit: Inherit via back propagation  FilterDenConstantOutMin=[]  FilterDenConstantOutMax=[]  PCopyOutDataTypeStr=Inherit: Inherit via back propagation  PCopyOutMin=[]  PCopyOutMax=[]  NCopyOutDataTypeStr=Inherit: Inherit via back propagation  NCopyOutMin=[]  NCopyOutMax=[]  IntegratorContinuousStateAttributes=''  IntegratorStateMustResolveToSignalObject=off  IntegratorRTWStateStorageClass=Auto  FilterContinuousStateAttributes=''  FilterStateMustResolveToSignalObject=off  FilterRTWStateStorageClass=Auto  ParallelPVariant=InternalParameters  IdealPVariant=Disabled  IVariant=InternalParameters  DVariant=Disabled  IntegratorVariant=Continuous  SatVariant=Disabled  AWVariant=Passthrough  PCopyVariant=Disabled  TRVariant=Disabled  FdbkBlocksVariant=Forward  IdealPFdbkVariant=Disabled  SatFdbkVariant=Disabled  DerivativeFilterVariant=Disabled  NVariant=Disabled  NCopyVariant=Disabled_SignalSpec  FilterICVariant=Disabled  IntegratorICVariant=InternalICs  ExternalResetVariant=Disabled  TRSumVariant=Passthrough  SumFdbkVariant=Disabled  SumVariant=Sum_PI  TsampFilterVariant=InternalTs  TsampNgainVariant=Passthrough  TsampIntegralVariant=Disabled_SignalSpec  ExternalSaturationOutDataTypeStr=Inherit: Same as second input  DerivativeSourceVariant=Disabled
  Product : Product
  Sum : Sum  Inputs=++|
  Sum1 : Sum  Inputs=+-
  Sum2 : Sum  Inputs=+-
  Transfer Fcn{1..5} (5 alike) : TransferFcn  Denominator=[0.00005 1]
  Vd_ref : Outport
  wires:
  Sum2/1 -> PID Controller2/1
  Product/1 -> Grid d-axis Current Control Loop/2, Sum1/1
  PID Controller2/1 -> Sum/2
  Divide/1 -> Gain/1
  [I_load_dc] -> Transfer Fcn5/1
  En_Injection/1 -> Product/1
  Sum/1 -> Product/2
  Constant2/1 -> Sum/1
  Transfer Fcn5/1 -> Divide/1
  [Vd_grid] -> Divide/3
  Constant3/1 -> Divide/2, DC-Link Voltage Control Loop/1, Sum2/1
  Sum1/1 -> PID Controller/1
  [Vd_grid] -> Découplage/3(Vd_grid)
  Vdc/1 -> Transfer Fcn3/1
  [iq_grid] -> Transfer Fcn1/1
  id_grid/1 -> Transfer Fcn4/1
  Découplage/1(Vd_ref) -> Transfer Fcn2/1
  PID Controller/1 -> Découplage/1(Vd)
  Transfer Fcn2/1 -> Vd_ref/1
  Transfer Fcn1/1 -> Découplage/2(iq_grid)
  Transfer Fcn3/1 -> DC-Link Voltage Control Loop/2, Sum2/2
  Transfer Fcn4/1 -> Sum1/2, Grid d-axis Current Control Loop/1

== system Projet_Final/Voltage Source Inverter (VSI)/GSC/Boucle iq_grid // Facteur de puissance ==
  note: Outer Control Level
  note: Inner Control Level
  note: iq_grid_ref
  note: Passage au mode injection
  En_Injection : Inport
  iq_grid : Inport  Port=2
  Q_mes : Inport  Port=3
  Constant3 : Constant  Value=0
  Grid q-axis Current Control Loop : Scope  NumInputPorts=2
  PID Controller1 : slpidlib/PID Controller  Controller=PI  Form=Parallel  TimeDomain=Continuous-time  UseExternalTs=off  SampleTime=-1  IntegratorMethod=Forward Euler  FilterMethod=Forward Euler  ControllerParametersSource=internal  P=kp_iq_grid  I=ki_iq_grid  UseKiTs=off  D=0  UseExternalDerivativeSource=off  N=100  UseFilter=on  TunerSelectOption=Transfer Function Based (PID Tuner App)  InitialConditionSource=internal  InitialConditionForIntegrator=0  InitialConditionForFilter=0  DifferentiatorICPrevScaledInput=0  ExternalReset=none  TrackingMode=off  Kt=1  LimitOutput=off  SatLimitsSource=internal  UpperSaturationLimit=inf  LowerSaturationLimit=-inf  LinearizeAsGain=on  AntiWindupMode=none  Kb=1  LimitIntegrator=off  UpperIntegratorSaturationLimit=inf  LowerIntegratorSaturationLimit=-inf  POutMin=[]  POutMax=[]  IOutMin=[]  IOutMax=[]  DOutMin=[]  DOutMax=[]  NOutMin=[]  NOutMax=[]  SumOutMin=[]  SumOutMax=[]  SaturationOutMin=[]  SaturationOutMax=[]  PParamMin=[]  PParamMax=[]  IParamMin=[]  IParamMax=[]  DParamMin=[]  DParamMax=[]  NParamMin=[]  NParamMax=[]  KbParamMin=[]  KbParamMax=[]  KtParamMin=[]  KtParamMax=[]  KbOutMin=[]  KbOutMax=[]  KtOutMin=[]  KtOutMax=[]  IntegratorOutMin=[]  IntegratorOutMax=[]  FilterOutMin=[]  FilterOutMax=[]  SumI1OutMin=[]  SumI1OutMax=[]  SumI2OutMin=[]  SumI2OutMax=[]  SumI3OutMin=[]  SumI3OutMax=[]  SumI4OutMin=[]  SumI4OutMax=[]  SumDOutMin=[]  SumDOutMax=[]  DifferentiatorOutMin=[]  DifferentiatorOutMax=[]  FilterDiffOutCoefMin=[]  FilterDiffOutCoefMax=[]  ReciprocalOutMin=[]  ReciprocalOutMax=[]  SumDenOutMin=[]  SumDenOutMax=[]  SumNumOutMin=[]  SumNumOutMax=[]  DivideOutMin=[]  DivideOutMax=[]  UdiffTsProdOutMin=[]  UdiffTsProdOutMax=[]  NTsProdOutMin=[]  NTsProdOutMax=[]  UintegralTsProdOutMin=[]  UintegralTsProdOutMax=[]  UngainTsProdOutMin=[]  UngainTsProdOutMax=[]  ClampingZeroOutDataTypeStr=Inherit: Inherit via back propagation  ClampingZeroOutMin=[]  ClampingZeroOutMax=[]  FilterDenConstantOutDataTypeStr=Inherit: Inherit via back propagation  FilterDenConstantOutMin=[]  FilterDenConstantOutMax=[]  PCopyOutDataTypeStr=Inherit: Inherit via back propagation  PCopyOutMin=[]  PCopyOutMax=[]  NCopyOutDataTypeStr=Inherit: Inherit via back propagation  NCopyOutMin=[]  NCopyOutMax=[]  IntegratorContinuousStateAttributes=''  IntegratorStateMustResolveToSignalObject=off  IntegratorRTWStateStorageClass=Auto  FilterContinuousStateAttributes=''  FilterStateMustResolveToSignalObject=off  FilterRTWStateStorageClass=Auto  ParallelPVariant=InternalParameters  IdealPVariant=Disabled  IVariant=InternalParameters  DVariant=Disabled  IntegratorVariant=Continuous  SatVariant=Disabled  AWVariant=Passthrough  PCopyVariant=Disabled  TRVariant=Disabled  FdbkBlocksVariant=Forward  IdealPFdbkVariant=Disabled  SatFdbkVariant=Disabled  DerivativeFilterVariant=Disabled  NVariant=Disabled  NCopyVariant=Disabled_SignalSpec  FilterICVariant=Disabled  IntegratorICVariant=InternalICs  ExternalResetVariant=Disabled  TRSumVariant=Passthrough  SumFdbkVariant=Disabled  SumVariant=Sum_PI  TsampFilterVariant=InternalTs  TsampNgainVariant=Passthrough  TsampIntegralVariant=Disabled_SignalSpec  ExternalSaturationOutDataTypeStr=Inherit: Same as second input  DerivativeSourceVariant=Disabled
  PID Controller3 : slpidlib/PID Controller  Controller=PI  Form=Parallel  TimeDomain=Continuous-time  UseExternalTs=off  SampleTime=-1  IntegratorMethod=Forward Euler  FilterMethod=Forward Euler  ControllerParametersSource=internal  P=kp_Q  I=ki_Q  UseKiTs=off  D=0  UseExternalDerivativeSource=off  N=100  UseFilter=on  TunerSelectOption=Transfer Function Based (PID Tuner App)  InitialConditionSource=internal  InitialConditionForIntegrator=0  InitialConditionForFilter=0  DifferentiatorICPrevScaledInput=0  ExternalReset=none  TrackingMode=off  Kt=1  LimitOutput=off  SatLimitsSource=internal  UpperSaturationLimit=inf  LowerSaturationLimit=-inf  LinearizeAsGain=on  AntiWindupMode=none  Kb=1  LimitIntegrator=off  UpperIntegratorSaturationLimit=inf  LowerIntegratorSaturationLimit=-inf  POutMin=[]  POutMax=[]  IOutMin=[]  IOutMax=[]  DOutMin=[]  DOutMax=[]  NOutMin=[]  NOutMax=[]  SumOutMin=[]  SumOutMax=[]  SaturationOutMin=[]  SaturationOutMax=[]  PParamMin=[]  PParamMax=[]  IParamMin=[]  IParamMax=[]  DParamMin=[]  DParamMax=[]  NParamMin=[]  NParamMax=[]  KbParamMin=[]  KbParamMax=[]  KtParamMin=[]  KtParamMax=[]  KbOutMin=[]  KbOutMax=[]  KtOutMin=[]  KtOutMax=[]  IntegratorOutMin=[]  IntegratorOutMax=[]  FilterOutMin=[]  FilterOutMax=[]  SumI1OutMin=[]  SumI1OutMax=[]  SumI2OutMin=[]  SumI2OutMax=[]  SumI3OutMin=[]  SumI3OutMax=[]  SumI4OutMin=[]  SumI4OutMax=[]  SumDOutMin=[]  SumDOutMax=[]  DifferentiatorOutMin=[]  DifferentiatorOutMax=[]  FilterDiffOutCoefMin=[]  FilterDiffOutCoefMax=[]  ReciprocalOutMin=[]  ReciprocalOutMax=[]  SumDenOutMin=[]  SumDenOutMax=[]  SumNumOutMin=[]  SumNumOutMax=[]  DivideOutMin=[]  DivideOutMax=[]  UdiffTsProdOutMin=[]  UdiffTsProdOutMax=[]  NTsProdOutMin=[]  NTsProdOutMax=[]  UintegralTsProdOutMin=[]  UintegralTsProdOutMax=[]  UngainTsProdOutMin=[]  UngainTsProdOutMax=[]  ClampingZeroOutDataTypeStr=Inherit: Inherit via back propagation  ClampingZeroOutMin=[]  ClampingZeroOutMax=[]  FilterDenConstantOutDataTypeStr=Inherit: Inherit via back propagation  FilterDenConstantOutMin=[]  FilterDenConstantOutMax=[]  PCopyOutDataTypeStr=Inherit: Inherit via back propagation  PCopyOutMin=[]  PCopyOutMax=[]  NCopyOutDataTypeStr=Inherit: Inherit via back propagation  NCopyOutMin=[]  NCopyOutMax=[]  IntegratorContinuousStateAttributes=''  IntegratorStateMustResolveToSignalObject=off  IntegratorRTWStateStorageClass=Auto  FilterContinuousStateAttributes=''  FilterStateMustResolveToSignalObject=off  FilterRTWStateStorageClass=Auto  ParallelPVariant=InternalParameters  IdealPVariant=Disabled  IVariant=InternalParameters  DVariant=Disabled  IntegratorVariant=Continuous  SatVariant=Disabled  AWVariant=Passthrough  PCopyVariant=Disabled  TRVariant=Disabled  FdbkBlocksVariant=Forward  IdealPFdbkVariant=Disabled  SatFdbkVariant=Disabled  DerivativeFilterVariant=Disabled  NVariant=Disabled  NCopyVariant=Disabled_SignalSpec  FilterICVariant=Disabled  IntegratorICVariant=InternalICs  ExternalResetVariant=Disabled  TRSumVariant=Passthrough  SumFdbkVariant=Disabled  SumVariant=Sum_PI  TsampFilterVariant=InternalTs  TsampNgainVariant=Passthrough  TsampIntegralVariant=Disabled_SignalSpec  ExternalSaturationOutDataTypeStr=Inherit: Same as second input  DerivativeSourceVariant=Disabled
  Product : Product
  Puissance réactive : Scope  NumInputPorts=2
  Subsystem : Subsystem
      settings: PortSchema="{\"entries\":[{\"content\":{\"sides\":[{\"content\":{\"connectorIds\":[\"In1\"]},\"type\":\"ConnectorPlacement.EquallySpacedRectSide\",\"uuid\":\"7d3af298-2f9f-475a-a651-f5eac2186357\"},{\"content\":{\"connectorIds\":[\"Out1\"],\"side\":\"RIGHT\"},\"type\":\"ConnectorPlacement.EquallySpacedRectSide\",\"uuid\":\"aa22588b-a98c-4a55-adf5-26eaad5d3043\"},{\"content\":{\"side\":\"TOP\"},\"type\":\"ConnectorPlacement.EquallySpacedRectSide\",\"uuid\":\"895af8ff-ad69-460f-8331-727a35d5d5ec\"},{\"content\":{\"connectorIds\":[\"In2\",\"In3\"],\"side\":\"BOTTOM\"},\"type\":\"ConnectorPlacement.EquallySpacedRectSide\",\"uuid\":\"a79db6ec-2ceb-4bca-883f-aa3bf861af08\"}]},\"type\":\"ConnectorPlacement.EquallySpacedConnector\",\"uuid\":\"f85c84fc-5e67-455b-b890-ed27a42cb9c3\"}],\"packageUris\":[\"http://schema.mathworks.com/mf0/Connector/R2020b\"],\"version\":\"1.0\"}"
  Sum : Sum  Inputs=+-
  Sum2 : Sum  Inputs=+-
  Transfer Fcn{1..4} (4 alike) : TransferFcn  Denominator=[0.00004 1]
  Vq_ref : Outport
  wires:
  Sum/1 -> PID Controller3/1
  Product/1 -> Grid q-axis Current Control Loop/1, Sum2/1
  Constant3/1 -> Sum/1, Puissance réactive/2
  En_Injection/1 -> Product/1
  PID Controller3/1 -> Product/2
  Sum2/1 -> PID Controller1/1
  [Vq_grid] -> Subsystem/3(Vq_grid)
  iq_grid/1 -> Transfer Fcn1/1
  Q_mes/1 -> Transfer Fcn2/1
  [id_grid] -> Transfer Fcn3/1
  Subsystem/1(Vq_ref) -> Transfer Fcn4/1
  PID Controller1/1 -> Subsystem/1(Vq)
  Transfer Fcn1/1 -> Sum2/2, Grid q-axis Current Control Loop/2
  Transfer Fcn2/1 -> Sum/2, Puissance réactive/1
  Transfer Fcn3/1 -> Subsystem/2(id_grid)
  Transfer Fcn4/1 -> Vq_ref/1

== system Projet_Final/Voltage Source Inverter (VSI)/GSC/Convertisseur Tension// PWM  ==
  abc_ref : Inport
  Divide3 : Product  Inputs=*/
  PWM Generator (2-Level) : spsPWMGenerator2LevelLib/PWM Generator (2-Level)  ModulatorType=Three-phase bridge (6 pulses)  ModulatorMode=Unsynchronized  Fc=Fc  Pc=90  nF=27  MinMax="[ -1  1 ]"  SamplingTechnique=Natural  ModulatingSignals=off  m=0.8  Freq=60  Phase=0  Ts=Ts  ShowCarrierOutport=off
  Scope : Scope
  Unit Delay1 : UnitDelay  SampleTime=Ts  HasFrameUpgradeWarning=on
  indiceM=33_(1/(fr*33)3 : Constant  Value=(Vdc_ref / 2)
  P1 : Outport
  wires:
  indiceM=33_(1/(fr*33)3/1 -> Divide3/2
  abc_ref/1 -> Divide3/1
  PWM Generator (2-Level)/1 -> P1/1
  Unit Delay1/1 -> PWM Generator (2-Level)/1, Scope/1
  Divide3/1 -> Unit Delay1/1
